simulink model "sample_rate21"  (Simulink 6.2)
settings: Solver=FixedStepDiscrete  StartTime=0.0  StopTime=1  RelTol=1e-3
libraries: dspsigops x2
settings Model: Creator=svenhoffmann  LastModifiedBy=svenhoffmann  ExtModeAutoUpdateStatusClock=off
settings DebuggingCC: SolverPrmCheckMsg=warning

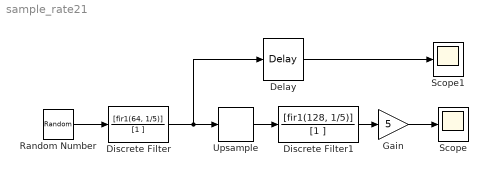
== system sample_rate21 ==
  Delay : dspsigops/Delay  dly_unit=Samples  delay=12  ic_detail=off  dif_ic_for_ch=off  dif_ic_for_dly=off  ic=0  reset_popup=None
  Discrete Filter : DiscreteFilter  Numerator=[fir1(64, 1/5)]  Denominator=[1 ]  SampleTime=-1
  Discrete Filter1 : DiscreteFilter  Numerator=[fir1(128, 1/5)]  Denominator=[1 ]  SampleTime=-1
  Gain : Gain  Gain=5
  Random Number : RandomNumber  SampleTime=1/1000
  Scope : Scope
  Scope1 : Scope
  Upsample : dspsigops/Upsample  N=5  phase=0  ic=0  mode=Maintain input frame size
  wires:
  Random Number/1 -> Discrete Filter/1
  Discrete Filter/1 -> Upsample/1, Delay/1
  Upsample/1 -> Discrete Filter1/1
  Discrete Filter1/1 -> Gain/1
  Gain/1 -> Scope/1
  Delay/1 -> Scope1/1
